simulink model "proj3_bf"  (Simulink 5.0)
settings: Solver=ode45  StartTime=0.0  StopTime=10  RelTol=1e-3
settings Model: LastModifiedBy=Frank Gloria

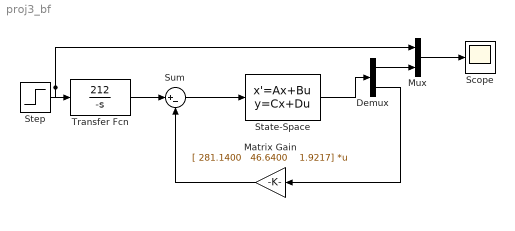
== system proj3_bf ==
  Demux : Demux  Outputs=2
  Matrix Gain : Gain  Orientation=left  Gain="[ 281.1400   46.6400    1.9217]"  Multiplication=Matrix(K*u) (u vector)  SaturateOnIntegerOverflow=on
  Mux : Mux  Inputs=2
  Scope : Scope
  State-Space : StateSpace  A=[1 1 0; -7 0 1;690 0 0]  B=[0;1;0]  C=[1 4 0; 1 0 0;0 1 0; 0 0 1]  D=[0; 0; 0; 0]
  Step : Step  Time=0  SampleTime=0
  Sum : Sum  Inputs=|+-  SaturateOnIntegerOverflow=on
  Transfer Fcn : TransferFcn  Numerator=[212]  Denominator=[-1 0]
  wires:
  Demux/2 -> Matrix Gain/1
  Step/1 -> Mux/1, Transfer Fcn/1
  State-Space/1 -> Demux/1
  Matrix Gain/1 -> Sum/2
  Sum/1 -> State-Space/1
  Demux/1 -> Mux/2
  Mux/1 -> Scope/1
  Transfer Fcn/1 -> Sum/1
